simulink model "DOOR"  (R2021b)
settings: Solver=FixedStepAuto  StartTime=0.0  StopTime=35  FixedStep=0.001  RelTol=1e-3  EnableMultiTasking=on
undefined symbols (not defined in the file): D10, D11, D12, D2, D4, D5, D7, D8, D9, PTA0, PTA2, PTB23, PTB9, PTC3, PTC4, PTD0, PTD2, PTD3
libraries: frdmk64flib x10, simulink x5
settings Model: SimulationMode=external  ExtModeTrigDuration=5  Creator=12268  LastModifiedBy=Aaron
settings SolverCC: AlgebraicLoopSolver=TrustRegion
settings OptimizationCC: EnhancedBackFolding=on  PassReuseOutputArgsAs=Individual arguments  ZeroExternalMemoryAtStartup=off  ZeroInternalMemoryAtStartup=off  MaxStackSize=64  OptimizeBlockOrder=speed  DifferentSizesBufferReuse=on  OptimizationCustomize=off  EfficientTunableParamExpr=on
settings DebuggingCC: ParameterTunabilityLossMsg=error  SFMachineParentedDataDiag=warning
settings HardwareCC: ProdBitPerPointer=32  ProdBitPerSizeT=32  ProdBitPerPtrDiffT=32  ProdLargestAtomicInteger=Long  ProdLargestAtomicFloat=Double  ProdWordSize=32  ProdHWDeviceType=ARM Compatible->ARM Cortex
settings SFSimCC: MATLABDynamicMemAlloc=off
settings RTWCC: Description=Embedded Coder  SystemTargetFile=ert.tlc  HardwareBoard=NXP FRDM-K64F  TLCOptions="-aInlineSetEventsForThisBaseRateFcn=TLC_FALSE -aSuppressMultiTaskScheduler=TLC_FALSE  -aRateBasedStepFcn=0"  TemplateMakefile=ert_default_tmf  Toolchain=GNU Tools for ARM Embedded Processors
settings CodeAppCC: ForceParamTrailComments=on  IgnoreCustomStorageClasses=off  OperatorAnnotations=on  SimulinkDataObjDesc=on  SFDataObjDesc=on  InsertBlockDesc=on
settings ERTTargetCC: ExtMode=on  ExtModeTransport=4  ExtModeMexFile=sendToCommService  ExtModeMexArgs='DOOR' 0

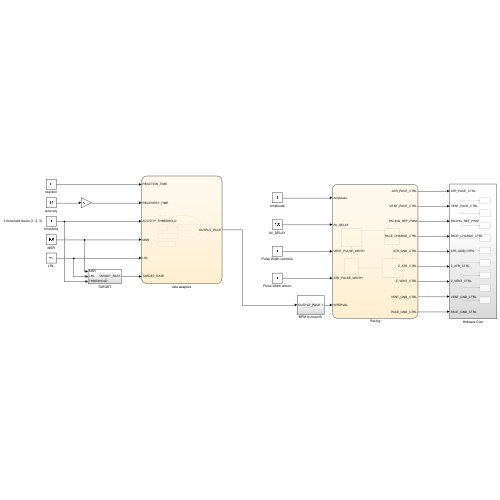
[thumbnail: Simulink's stored preview of the top-level diagram]
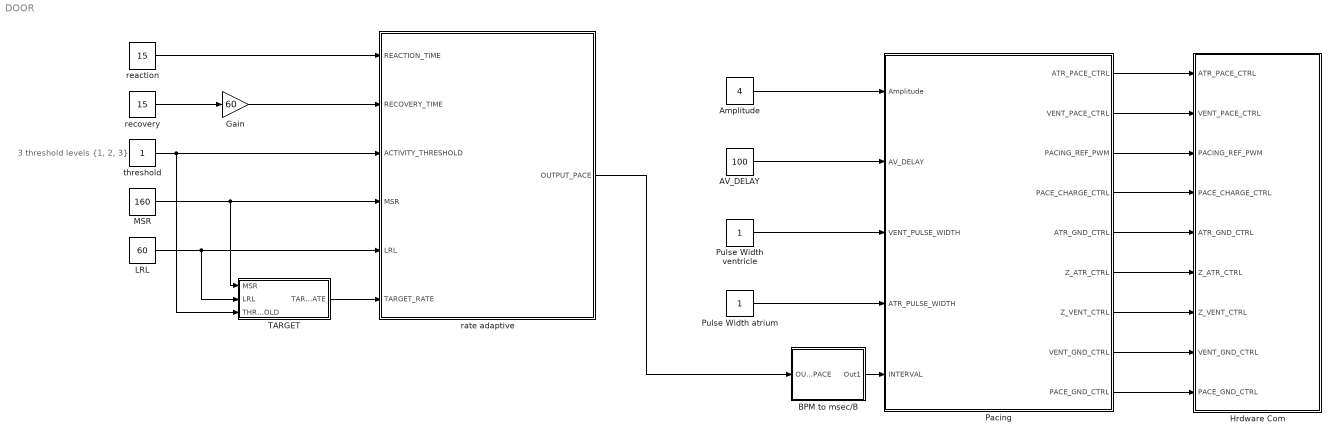
== system DOOR ==
  note: 3 threshold levels {1, 2, 3}
  AV_DELAY : Constant  Value=100  OutDataTypeStr=uint16
  Amplitude : Constant  Value=4  OutDataTypeStr=double
  "BPM to msec/B " : Subsystem
  Gain : Gain  Gain=60
  Hrdware Com : Subsystem
  LRL : Constant  Value=60
  MSR : Constant  Value=160
  Pacing : Stateflow chart  TreatAsAtomicUnit=on
      settings: PortSchema="{\"entries\":[{\"content\":{\"sides\":[{\"content\":{\"connectorIds\":[\"In1\",\"In5\",\"In2\",\"In3\",\"In4\"]},\"type\":\"ConnectorPlacement.EquallySpacedRectSide\",\"uuid\":\"72970874-2a7f-4f54-9c96-49c3612305c0\"},{\"content\":{\"connectorIds\":[\"Out1\",\"Out2\",\"Out3\",\"Out4\",\"Out5\",\"Out6\",\"Out7\",\"Out8\",\"Out9\"],\"side\":\"RIGHT\"},\"type\":\"ConnectorPlacement.EquallySpacedRectSide\",\"uuid\":\"785d6d73-c00d-4bb6-bac4-9062a7713100\"},{\"content\":{\"connectorIds\":[],\"side\":\"TOP\"},\"type\":\"ConnectorPlacement.EquallySpacedRectSide\",\"uuid\":\"f7c58201-4adc-48cf-bf7a-118db90373b1\"}]},\"type\":\"ConnectorPlacement.EquallySpacedConnector\",\"uuid\":\"33960bc4-ecd9-4e8c-b37b-5f7b6e376475\"}],\"packageUris\":[\"http://schema.mathworks.com/mf0/Connector/R2020b\"],\"version\":\"1.0\"}"
  Pulse Width atrium : Constant  OutDataTypeStr=uint16
  Pulse Width ventricle : Constant  OutDataTypeStr=uint16
  TARGET : Subsystem
  rate adaptive : Stateflow chart  TreatAsAtomicUnit=on
      settings: PortSchema="{\"entries\":[{\"content\":{\"sides\":[{\"content\":{\"connectorIds\":[\"In3\",\"In4\",\"In5\",\"In1\",\"In2\",\"In6\"]},\"type\":\"ConnectorPlacement.EquallySpacedRectSide\",\"uuid\":\"d3aa46b7-da68-4733-bd03-102d604fce17\"},{\"content\":{\"connectorIds\":[\"Out1\"],\"side\":\"RIGHT\"},\"type\":\"ConnectorPlacement.EquallySpacedRectSide\",\"uuid\":\"afbb636e-6b76-41fa-bb75-ca0d3f63044e\"},{\"content\":{\"connectorIds\":[],\"side\":\"TOP\"},\"type\":\"ConnectorPlacement.EquallySpacedRectSide\",\"uuid\":\"40571637-2e0f-45fd-89f0-6c332ecbd683\"}]},\"type\":\"ConnectorPlacement.EquallySpacedConnector\",\"uuid\":\"5e4e3dcb-fc0d-40cc-8fd4-4ca115cadd01\"}],\"packageUris\":[\"http://schema.mathworks.com/mf0/Connector/R2020b\"],\"version\":\"1.0\"}"
  reaction : Constant  Value=15  OutDataTypeStr=double
  recovery : Constant  Value=15  OutDataTypeStr=double
  threshold : Constant  OutDataTypeStr=single
  wires:
  Pacing/1(ATR_PACE_CTRL) -> Hrdware Com/1(ATR_PACE_CTRL)
  Amplitude/1 -> Pacing/1(Amplitude)
  Pacing/9(PACE_GND_CTRL) -> Hrdware Com/9(PACE_GND_CTRL)
  Pacing/3(PACING_REF_PWM) -> Hrdware Com/3(PACING_REF_PWM)
  Pacing/2(VENT_PACE_CTRL) -> Hrdware Com/2(VENT_PACE_CTRL)
  Pacing/4(PACE_CHARGE_CTRL) -> Hrdware Com/4(PACE_CHARGE_CTRL)
  Pacing/5(ATR_GND_CTRL) -> Hrdware Com/5(ATR_GND_CTRL)
  Pacing/6(Z_ATR_CTRL) -> Hrdware Com/6("Z_ATR_CTRL ")
  Pacing/7(Z_VENT_CTRL) -> Hrdware Com/7("Z_VENT_CTRL ")
  Pacing/8(VENT_GND_CTRL) -> Hrdware Com/8(VENT_GND_CTRL)
  Pulse Width ventricle/1 -> Pacing/2(VENT_PULSE_WIDTH)
  "BPM to msec/B "/1(Out1) -> Pacing/4(INTERVAL)
  AV_DELAY/1 -> Pacing/5(AV_DELAY)
  Pulse Width atrium/1 -> Pacing/3(ATR_PULSE_WIDTH)
  TARGET/1(TARGET_RATE) -> rate adaptive/6(TARGET_RATE)
  rate adaptive/1(OUTPUT_PACE) -> "BPM to msec/B "/1(OUTPUT_PACE)
  MSR/1 -> TARGET/1(MSR), rate adaptive/1(MSR)
  reaction/1 -> rate adaptive/3(REACTION_TIME)
  recovery/1 -> Gain/1
  threshold/1 -> TARGET/3(THRESHOLD), rate adaptive/5(ACTIVITY_THRESHOLD)
  Gain/1 -> rate adaptive/4(RECOVERY_TIME)
  LRL/1 -> rate adaptive/2(LRL), TARGET/2(LRL)

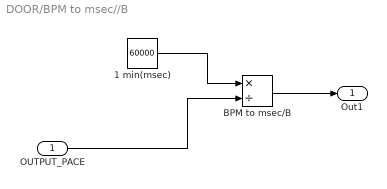
== system DOOR/BPM to msec//B  ==
  OUTPUT_PACE : Inport
  1 min(msec) : Constant  Value=60000  OutDataTypeStr=double
  "BPM to msec/B " : Product  Inputs=*/  OutDataTypeStr=uint16  RndMeth=Nearest
  Out1 : Outport  OutDataTypeStr=uint16
  wires:
  1 min(msec)/1 -> "BPM to msec/B "/1
  "BPM to msec/B "/1 -> Out1/1
  OUTPUT_PACE/1 -> "BPM to msec/B "/2

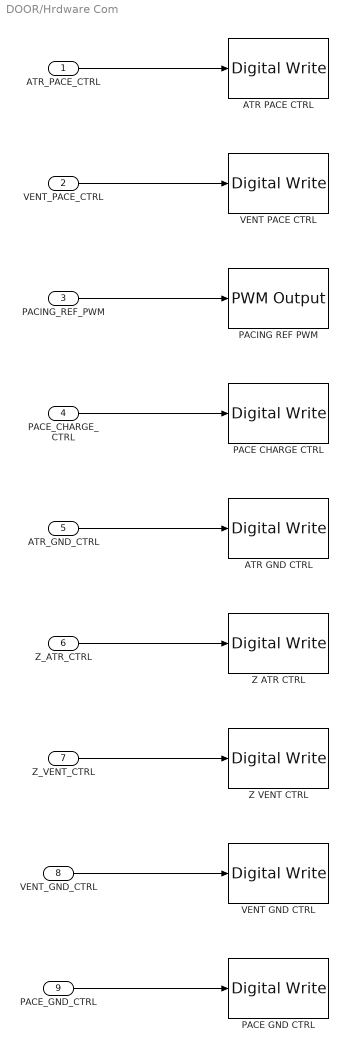
== system DOOR/Hrdware Com ==
  ATR_PACE_CTRL : Inport
  VENT_PACE_CTRL : Inport  Port=2
  PACING_REF_PWM : Inport  Port=3
  PACE_CHARGE_CTRL : Inport  Port=4
  ATR_GND_CTRL : Inport  Port=5
  "Z_ATR_CTRL " : Inport  Port=6
  "Z_VENT_CTRL " : Inport  Port=7
  VENT_GND_CTRL : Inport  Port=8
  PACE_GND_CTRL : Inport  Port=9
  "ATR GND CTRL " : frdmk64flib/Digital Write  Whichpin=PTD2 (D11)
  ATR PACE CTRL : frdmk64flib/Digital Write  Whichpin=PTA0 (D8)
  PACE CHARGE CTRL : frdmk64flib/Digital Write  Whichpin=PTB9 (D2)
  PACE GND CTRL : frdmk64flib/Digital Write  Whichpin=PTD0 (D10)
  PACING REF PWM : frdmk64flib/PWM Output  Whichpin=PTA2 (D5)  InitialFrequency=2000  InitialDutyCycle=0
  VENT GND CTRL : frdmk64flib/Digital Write  Whichpin=PTD3 (D12)
  VENT PACE CTRL : frdmk64flib/Digital Write  Whichpin=PTC4 (D9)
  "Z ATR CTRL " : frdmk64flib/Digital Write  Whichpin=PTB23 (D4)
  "Z VENT CTRL " : frdmk64flib/Digital Write  Whichpin=PTC3 (D7)
  wires:
  ATR_PACE_CTRL/1 -> ATR PACE CTRL/1
  VENT_PACE_CTRL/1 -> VENT PACE CTRL/1
  PACING_REF_PWM/1 -> PACING REF PWM/1
  PACE_CHARGE_CTRL/1 -> PACE CHARGE CTRL/1
  ATR_GND_CTRL/1 -> "ATR GND CTRL "/1
  "Z_ATR_CTRL "/1 -> "Z ATR CTRL "/1
  "Z_VENT_CTRL "/1 -> "Z VENT CTRL "/1
  VENT_GND_CTRL/1 -> VENT GND CTRL/1
  PACE_GND_CTRL/1 -> PACE GND CTRL/1

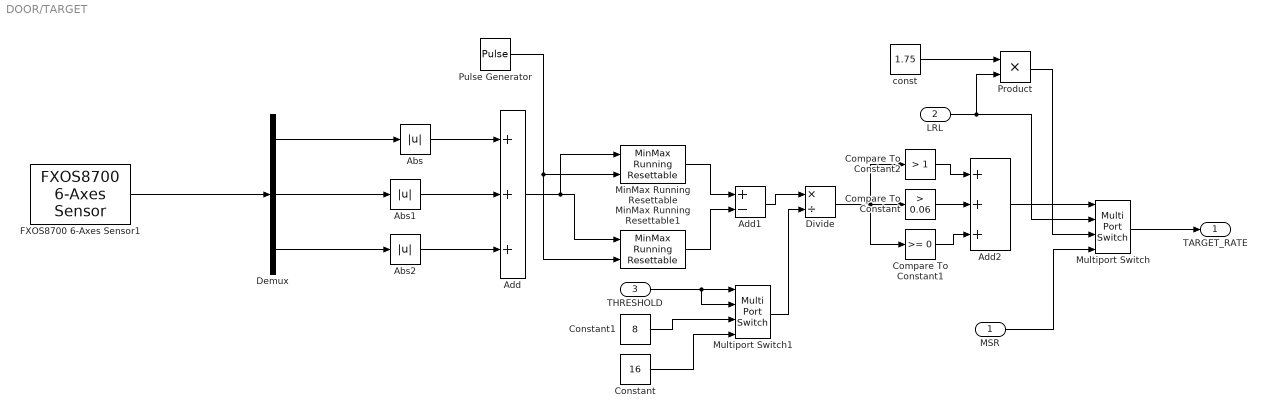
== system DOOR/TARGET ==
  MSR : Inport
  LRL : Inport  Port=2
  THRESHOLD : Inport  Port=3
  Abs : Abs
  Abs1 : Abs
  Abs2 : Abs
  Add : Sum  Inputs=+++
  Add1 : Sum  Inputs=+-
  Add2 : Sum  Inputs=+++
  Compare To Constant : simulink/Logic and Bit Operations/Compare To Constant  relop=>  const=0.06  OutDataTypeStr=uint8
  Compare To Constant1 : simulink/Logic and Bit Operations/Compare To Constant  relop=>=  const=0  OutDataTypeStr=uint8
  Compare To Constant2 : simulink/Logic and Bit Operations/Compare To Constant  relop=>  const=1  OutDataTypeStr=uint8
  Constant : Constant  Value=16  OutDataTypeStr=single
  Constant1 : Constant  Value=8  OutDataTypeStr=single
  Demux : Demux  Outputs=3
  Divide : Product  Inputs=*/
  FXOS8700 6-Axes Sensor1 : frdmk64flib/FXOS8700 6-Axes Sensor  Activesensor=Accelerometer only  ODR=800Hz  HybridODR=400Hz  Accelfullrange=-2g to +2g  SampleTime=-1
  MinMax Running Resettable : simulink/Math Operations/MinMax Running Resettable  Function=max  vinit=1
  MinMax Running Resettable1 : simulink/Math Operations/MinMax Running Resettable  Function=min  vinit=1
  Multiport Switch : MultiPortSwitch  OutDataTypeStr=double
  Multiport Switch1 : MultiPortSwitch
  Product : Product
  Pulse Generator : DiscretePulseGenerator  PulseType=Time based  PulseWidth=2.5
  const : Constant  Value=1.75
  TARGET_RATE : Outport
  wires:
  Compare To Constant/1 -> Add2/2
  Multiport Switch/1 -> TARGET_RATE/1
  Compare To Constant1/1 -> Add2/3
  Add2/1 -> Multiport Switch/1
  LRL/1 -> Product/2, Multiport Switch/2
  Product/1 -> Multiport Switch/3
  Abs2/1 -> Add/3
  Add/1 -> MinMax Running Resettable1/1, MinMax Running Resettable/1
  MinMax Running Resettable1/1 -> Add1/2
  Demux/2 -> Abs1/1
  Demux/3 -> Abs2/1
  Compare To Constant2/1 -> Add2/1
  MinMax Running Resettable/1 -> Add1/1
  Demux/1 -> Abs/1
  Pulse Generator/1 -> MinMax Running Resettable1/2, MinMax Running Resettable/2
  Abs/1 -> Add/1
  Abs1/1 -> Add/2
  FXOS8700 6-Axes Sensor1/1 -> Demux/1
  MSR/1 -> Multiport Switch/4
  const/1 -> Product/1
  Divide/1 -> Compare To Constant/1, Compare To Constant2/1, Compare To Constant1/1
  Add1/1 -> Divide/1
  Multiport Switch1/1 -> Divide/2
  THRESHOLD/1 -> Multiport Switch1/2, Multiport Switch1/1
  Constant/1 -> Multiport Switch1/4
  Constant1/1 -> Multiport Switch1/3

== stateflow chart DOOR/rate adaptive ==
  state start
    entry:
    OUTPUT_PACE = LRL;
  state IDLE
  state increase_pace
    entry:
    OUTPUT_PACE = OUTPUT_PACE + increment;
  state calculate_increment
    entry:
    increment = 2.5*(TARGET_RATE-OUTPUT_PACE) / REACTION_TIME;
  state calculate_decrement
    entry:
    decrement = (OUTPUT_PACE - TARGET_RATE) / RECOVERY_TIME;
  state decrease_pace
    entry:
    OUTPUT_PACE = OUTPUT_PACE - decrement;
  (default) -> start
  increase_pace -> IDLE [order 1] : [OUTPUT_PACE == TARGET_RATE]
  start -> IDLE
  calculate_increment -> increase_pace
  decrease_pace -> IDLE : after(500,msec)
  IDLE -> calculate_increment [order 1] : [TARGET_RATE > OUTPUT_PACE]
  IDLE -> calculate_decrement [order 2] : [TARGET_RATE < OUTPUT_PACE]
  increase_pace -> calculate_decrement [order 3] : [TARGET_RATE < OUTPUT_PACE]
  increase_pace -> increase_pace [order 2] : after(1,sec)
  calculate_decrement -> decrease_pace
  data: MSR input double; LRL input double; REACTION_TIME input double; RECOVERY_TIME input double; ACTIVITY_THRESHOLD input single; OUTPUT_PACE output double; TARGET_RATE input double; decrement local double; increment local double

== stateflow chart DOOR/Pacing ==
  state A_Charging
    entry:
    PACE_GND_CTRL=true;
    ATR_PACE_CTRL=false;
    VENT_PACE_CTRL=false;
    PACING_REF_PWM=uint8(Amplitude*20);
    PACE_CHARGE_CTRL=true;
    Z_ATR_CTRL=false;
    Z_VENT_CTRL=false;
    VENT_GND_CTRL=true;
    ATR_GND_CTRL=false;
  state A_Pacing
    entry:
    PACE_CHARGE_CTRL=false;
    PACE_GND_CTRL=true;
    ATR_GND_CTRL=false;
    Z_ATR_CTRL=false;
    Z_VENT_CTRL=false;
    VENT_GND_CTRL=false;
    VENT_PACE_CTRL=false;
    ATR_PACE_CTRL=true;
  state V_Pacing
    entry:
    PACE_CHARGE_CTRL=false;
    PACE_GND_CTRL=true;
    ATR_GND_CTRL=false;
    Z_ATR_CTRL=false;
    Z_VENT_CTRL=false;
    VENT_GND_CTRL=false;
    VENT_PACE_CTRL=true;
    ATR_PACE_CTRL=false;
  state V_Charging
    entry:
    PACE_GND_CTRL=true;
    ATR_PACE_CTRL=false;
    VENT_PACE_CTRL=false;
    PACING_REF_PWM=uint8(Amplitude*20);
    PACE_CHARGE_CTRL=true;
    Z_ATR_CTRL=false;
    Z_VENT_CTRL=false;
    VENT_GND_CTRL=false;
    ATR_GND_CTRL=true;
  (default) -> A_Charging
  A_Charging -> A_Pacing : after(INTERVAL-VENT_PULSE_WIDTH-AV_DELAY, msec)
  A_Pacing -> V_Charging : after(ATR_PULSE_WIDTH,msec)
  V_Pacing -> A_Charging : after(VENT_PULSE_WIDTH,msec)
  V_Charging -> V_Pacing : after(AV_DELAY-ATR_PULSE_WIDTH,msec)
  data: ATR_PACE_CTRL output boolean; VENT_PACE_CTRL output boolean; PACING_REF_PWM output uint8; Amplitude input double; PACE_CHARGE_CTRL output boolean; ATR_GND_CTRL output boolean; Z_ATR_CTRL output boolean; Z_VENT_CTRL output boolean; VENT_GND_CTRL output boolean; PACE_GND_CTRL output boolean; VENT_PULSE_WIDTH input uint16; ATR_PULSE_WIDTH input uint16; INTERVAL input uint16; AV_DELAY input uint16
